simulink model "Motor_Pump"  (R2019b)
settings: Solver=VariableStepAuto  StartTime=0.0  StopTime=1.5  RelTol=1e-6  AbsTol=1e-9
InitFcn:
  | kp2 = 8000;  % [Nm/rad]
  | k1  = 1200;   % [Nm/rad]
  | k2  = 2000;   % [Nm/rad]
  | 
  | Jp2 = 4.5;     % [kgm^2]
  | Jp3 = 2;        % [kgm^2]
  | J1   = 1.5;     % [kgm^2]
  | J2   = 0.5;     % [kgm^2]
  | J3   = 1.0;     % [kgm^2]
  | J4   = 2.0;     % [kgm^2]
  | 
  | 
settings Model: Creator=sulaymon.eshkabilov  LastModifiedBy=sulaymon.eshkabilov

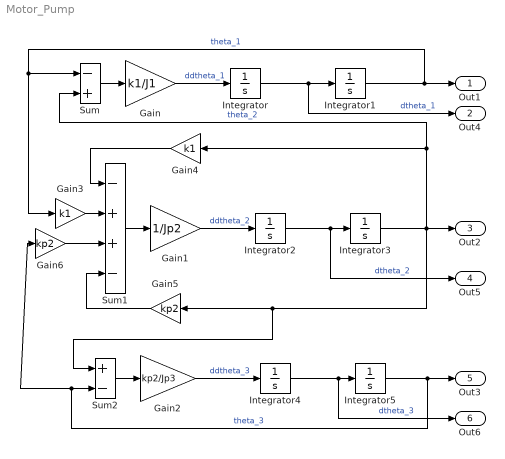
== system Motor_Pump ==
  Gain : Gain  Gain=k1/J1
  Gain1 : Gain  Gain=1/Jp2
  Gain2 : Gain  Gain=kp2/Jp3
  Gain3 : Gain  Gain=k1
  Gain4 : Gain  Gain=k1
  Gain5 : Gain  Gain=kp2
  Gain6 : Gain  Gain=kp2
  Integrator{,2..5} (5 alike) : Integrator
  Integrator1 : Integrator  InitialCondition=0.005
  Sum : Sum  Inputs=-+
  Sum1 : Sum  Inputs=-++-
  Sum2 : Sum  Inputs=+-
  Out1 : Outport
  Out4 : Outport  Port=2
  Out2 : Outport  Port=3
  Out5 : Outport  Port=4
  Out3 : Outport  Port=5
  Out6 : Outport  Port=6
  wires:
  Integrator2/1 -> Integrator3/1, Out5/1  "dtheta_2"
  Integrator/1 -> Out4/1, Integrator1/1  "dtheta_1"
  Integrator4/1 -> Integrator5/1, Out6/1  "dtheta_3"
  Gain2/1 -> Integrator4/1  "ddtheta_3"
  Gain1/1 -> Integrator2/1  "ddtheta_2"
  Gain/1 -> Integrator/1  "ddtheta_1"
  Sum2/1 -> Gain2/1
  Sum1/1 -> Gain1/1
  Sum/1 -> Gain/1
  Integrator1/1 -> Out1/1, Sum/1, Gain3/1  "theta_1"
  Integrator3/1 -> Out2/1, Sum/2, Gain4/1, Sum2/1, Gain5/1  "theta_2"
  Integrator5/1 -> Out3/1, Gain6/1, Sum2/2  "theta_3"
  Gain3/1 -> Sum1/2
  Gain4/1 -> Sum1/1
  Gain5/1 -> Sum1/4
  Gain6/1 -> Sum1/3
